simulink model "Model_GBXCluctchOpt_V5"  (R2024b)
settings: Solver=VariableStepAuto  StartTime=0.0  StopTime=552  RelTol=1e-5
undefined symbols (not defined in the file): Bdy_facCoG_C, Bdy_facTireFric_C, Bdy_lenRadiusWheel_C, Bdy_lenWheelBase_C, Bdy_lenZCoG_C, Bdy_mEquivalentJ_C, Bdy_mVeh_C, Bdy_vsqr2frc_C, Drv_kmh2gradtqDriver_C, Drv_kmh2tqDriver_C, Edr_pwr_LossMap_AXIS, Edr_pwrInverterLosses_MAP, Edr_pwrMachineLosses_MAP, Edr_rpm_InvLossMap_AXIS, Edr_rpm_MachLossMap_AXIS, Edr_rpm_MaxMinTq_AXIS, Edr_rpmMax_C, Edr_tq_MachLossMap_AXIS, Edr_tqEffMax_CUR, Env_facSlope_WLTC_CUR, Env_facSlopeBAB185_CUR, Env_facSlopeCrossCountry_CUR, Env_kmhDesBAB185_CUR, Env_kmhDesCrossCountry_CUR, Env_vVehDes_NEDC_kmh, Env_vVehDes_WLTC_kmh, Env_vVehTime_NEDC_s, Env_vVehTime_WLTC_s, Gbx_facGbxRatioRe_C, Ice_derfacLoadDecrease_MAP, Ice_derfacLoadIncrease_MAP, Ice_etaLam_CUR, Ice_facEtaCocMax_MAP, Ice_facFuelEnRich_MAP, Ice_KUMSRL_C, Ice_Lambda_AXIS, Ice_relLoad2relTqOptIgnLamOne_MAP, Ice_relLoad_AXIS, Ice_relLoad_LoadDyn_AXIS, Ice_relLoad_Max_CUR, Ice_relTq_AXIS, Ice_relTqInr2TqInr_C, Ice_relTqOptIgnLamOne2relLoad_MAP, Ice_rpm_AXIS, Ice_rpm_LoadDyn_AXIS, Ice_rpm_relLoadMax_AXIS, Ice_tqLossesIce_MAP, Pnt_capBat_C, Pnt_facSocBatOcv_AXIS, Pnt_facSocInit_C, Pnt_iBatChrgMax_C, Pnt_iBatDisChrgMax_C, Pnt_resBatInner_C, Pnt_uBatMax_C, Pnt_uBatMin_C, Pnt_uBatOcv_CUR, Vco_flgEdrExists_CFG, Vco_flgIceCluAlwClosed_CFG, Vco_flgIceExists_CFG
libraries: simulink x7, simulink_extras x6
(part 1 of 3)
settings Model: Creator=Georg  LastModifiedBy=Raj Srivastava
settings SolverCC: AlgebraicLoopSolver=TrustRegion
settings DebuggingCC: IgnoredZcDiagnostic=none  UnconnectedInputMsg=warning  UnconnectedOutputMsg=warning  UnconnectedLineMsg=warning
settings HardwareCC: ProdHWDeviceType=AMD->x86-64 (Windows64)
settings ModelReferenceCC: EnableRefExpFcnMdlSchedulingChecks=on
settings RTWCC: GPUComputeCapability=3.5  DLArmComputeVersion=19.05

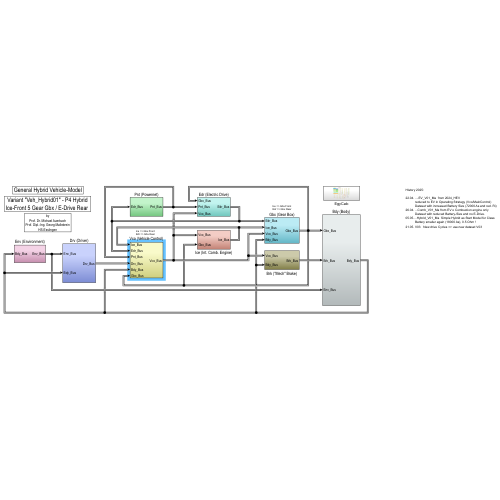
[thumbnail: Simulink's stored preview of the top-level diagram]
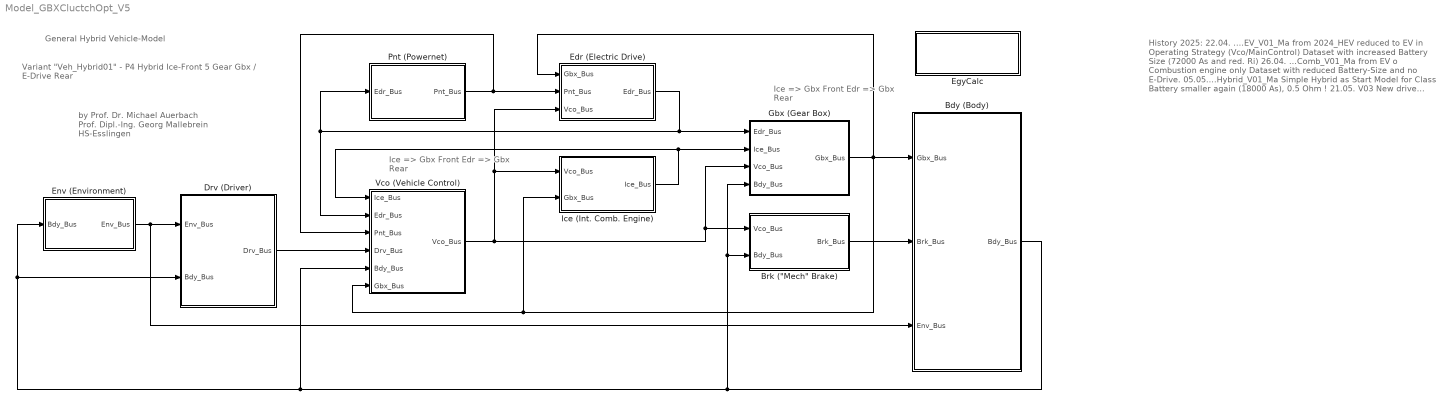
== system Model_GBXCluctchOpt_V5 ==
  note: History 2025:
      |
      | 22.04. ....EV_V01_Ma  from 2024_HEV
      |            reduced to EV in Operating Strategy (Vco/MainControl)
      |            Dataset with increased Battery Size (72000 As and red. Ri)
      | 26.04. ...Comb_V01_Ma from EV o Combustion engine only
      |            Dataset with reduced Battery-Size and no E-Drive.
      | 05.05....Hybrid_V01_Ma  Simple Hybrid as Start Model for Class
      |            Battery smaller again (18000 As), 0.5 Ohm !
      | 21.05. V03   New drive Cycles => use new dataset V03
  note: General Hybrid Vehicle-Model
  note: Ice => Gbx Front
      | Edr => Gbx Rear
  note: Ice => Gbx Front
      | Edr => Gbx Rear
  note: by
      | Prof. Dr. Michael Auerbach
      | Prof. Dipl.-Ing. Georg Mallebrein
      | HS-Esslingen
  note: Variant "Veh_Hybrid01" - P4 Hybrid
      | Ice-Front 5 Gear Gbx / E-Drive Rear
  Bdy (Body) : Subsystem
  "Brk (\"Mech\" Brake)" : Subsystem
  Drv (Driver) : Subsystem
  Edr (Electric Drive) : Subsystem
  EgyCalc : Subsystem
  Env (Environment) : Subsystem
  Gbx (Gear Box) : Subsystem
  Ice (Int. Comb. Engine) : Subsystem
  Pnt (Powernet) : Subsystem
  Vco (Vehicle Control) : Subsystem
  wires:
  Gbx (Gear Box)/1(Gbx_Bus) -> Edr (Electric Drive)/1(Gbx_Bus), Bdy (Body)/1(Gbx_Bus), Ice (Int. Comb. Engine)/2(Gbx_Bus), Vco (Vehicle Control)/6(Gbx_Bus)
  "Brk (\"Mech\" Brake)"/1(Brk_Bus) -> Bdy (Body)/2(Brk_Bus)
  Pnt (Powernet)/1(Pnt_Bus) -> Edr (Electric Drive)/2(Pnt_Bus), Vco (Vehicle Control)/3(Pnt_Bus)
  Edr (Electric Drive)/1(Edr_Bus) -> Vco (Vehicle Control)/2(Edr_Bus), Pnt (Powernet)/1(Edr_Bus), Gbx (Gear Box)/1(Edr_Bus)
  Ice (Int. Comb. Engine)/1(Ice_Bus) -> Vco (Vehicle Control)/1(Ice_Bus), Gbx (Gear Box)/2(Ice_Bus)
  Vco (Vehicle Control)/1(Vco_Bus) -> Edr (Electric Drive)/3(Vco_Bus), Ice (Int. Comb. Engine)/1(Vco_Bus), Gbx (Gear Box)/3(Vco_Bus), "Brk (\"Mech\" Brake)"/1(Vco_Bus)
  Drv (Driver)/1(Drv_Bus) -> Vco (Vehicle Control)/4(Drv_Bus)
  Env (Environment)/1(Env_Bus) -> Bdy (Body)/3(Env_Bus), Drv (Driver)/1(Env_Bus)
  Bdy (Body)/1(Bdy_Bus) -> Env (Environment)/1(Bdy_Bus), Drv (Driver)/2(Bdy_Bus), Vco (Vehicle Control)/5(Bdy_Bus), "Brk (\"Mech\" Brake)"/2(Bdy_Bus), Gbx (Gear Box)/4(Bdy_Bus)

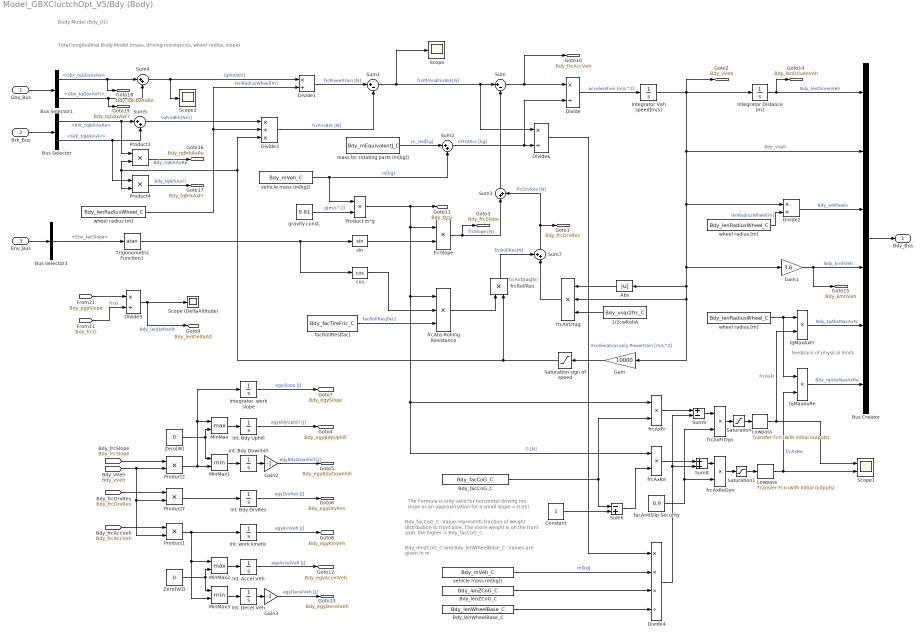
== system Model_GBXCluctchOpt_V5/Bdy (Body) ==
  note: feedback of physical limits
  note: Bdy_facCoG_C: Value represents fraction of weight distribution to front axle. The more weight is on the front axle, the higher is Bdy_facCoG_C.
  note: Total longitudinal Body Model (mass, driving resistances, wheel radius, slope)
  note: Bdy_lenZCoG_C and Bdy_lenWheelBase_C: Values are given in m
  note: The Formula is only valid for horizontal driving (no slope or an approximation for a small slope < 0.05)
  note: Body Model (Bdy_01)
  Gbx_Bus : Inport
  Brk_Bus : Inport  Port=2
  Env_Bus : Inport  Port=3
  " wheel radius [m]  " : Constant  Value=Bdy_lenRadiusWheel_C
  1/2cwRohA : Constant  Value=Bdy_vsqr2frc_C
  Abs : Abs  SaturateOnIntegerOverflow=off
  Bdy_facCoG_C : Constant  Value=Bdy_facCoG_C
  Bdy_lenWheelBase_C : Constant  Value=Bdy_lenWheelBase_C
  Bdy_lenZCoG_C : Constant  Value=Bdy_lenZCoG_C
  Bus Creator : BusCreator  Inputs=6
  Bus Selector : BusSelector  OutputSignals=Brk_tqBrkAxRe,Brk_tqBrkAxFr
  Bus Selector1 : BusSelector  OutputSignals=Gbx_tqGbxAxRe,Gbx_tqGbxAxFr
  Bus Selector3 : BusSelector  OutputSignals=Env_facSlope
  Constant : Constant
  Divide{,1..2,5..6} (5 alike) : Product  Inputs=*/
  Divide3 : Product  Inputs=*/*
  Divide4 : Product  Inputs=***/
  Gain : Gain  Gain=10000
  Gain1 : Gain  Gain=3.6
  Gain2 : Gain  Gain=-1
  Gain3 : Gain  Gain=-1
  Int. Accel Veh : Integrator
  Int. Bdy Downhill : Integrator
  Int. Bdy DrvRes : Integrator
  Int. Bdy Uphill : Integrator
  Int. Decel Veh : Integrator
  Int. work kinetic : Integrator
  Integrator Distance [m] : Integrator  InitialCondition=1E-10
  Integrator Veh speed[m/s] : Integrator
  Integrator  work slope : Integrator
  Lowpass : simulink_extras/Additional Linear/Transfer Fcn (with initial outputs)  N=[1]  D=[0.000001 1]  Y0=1  U0=0
  "Lowpass " : simulink_extras/Additional Linear/Transfer Fcn (with initial outputs)  N=[1]  D=[0.000001 1]  Y0=1  U0=0
  MinMax : MinMax  Function=max  Inputs=2  ZeroCross=off
  MinMax1 : MinMax  Inputs=2  ZeroCross=off
  MinMax2 : MinMax  Function=max  Inputs=2  ZeroCross=off
  MinMax3 : MinMax  Inputs=2  ZeroCross=off
  Product m*g : Product
  Product{1..4,7} (5 alike) : Product
  Saturation : Saturate  UpperLimit=inf  LowerLimit=0
  Saturation sign of speed : Saturate  UpperLimit=1  LowerLimit=-1
  Saturation1 : Saturate  UpperLimit=inf  LowerLimit=0
  Scope : Scope
  "Scope (DeltaAltitude) " : Scope
  Scope1 : Scope  NumInputPorts=2
  Scope2 : Scope
  Sum : Sum  Inputs=|+-
  Sum1 : Sum  Inputs=|+-
  Sum{2..5} (4 alike) : Sum  Inputs=|++
  Sum6 : Sum  Inputs=-+
  Sum7 : Sum  Inputs=++|
  Sum8 : Sum
  Sum9 : Sum  Inputs=+-
  Trigonometric Function1 : Trigonometry  Operator=atan
  Zero[W] : Constant  Value=0
  Zero[W]1 : Constant  Value=0
  cos : Trigonometry  Operator=cos
  facAntiSlip Security : Constant  Value=0.9
  facRollRes[fac] : Constant  Value=Bdy_facTireFric_C
  frcAbs Rolling Resistance : Product  Inputs=3
  frcAirDrag : Product  Inputs=3
  frcAxFr : Product
  frcAxFrDyn : Product
  frcAxRe : Product
  frcAxReDyn : Product
  frcRollRes : Product
  frcSlope : Product
  gravity const. : Constant  Value=9.81
  mass for rotating parts (m[kg]) : Constant  Value=Bdy_mEquivalentJ_C
  sin : Trigonometry
  tqMaxAxFr : Product
  tqMaxAxRe : Product
  vehicle mass (m[kg]) : Constant  Value=Bdy_mVeh_C
  "vehicle mass (m[kg]) " : Constant  Value=Bdy_mVeh_C
  wheel radius [m] : Constant  Value=Bdy_lenRadiusWheel_C
  "wheel radius [m] " : Constant  Value=Bdy_lenRadiusWheel_C
  Bdy_Bus : Outport  VectorParamsAs1DForOutWhenUnconnected=off
  tag scope: Bdy_egyAccelVeh=global, Bdy_egyBdyDownhill=global, Bdy_egyBdyUphill=global, Bdy_egyDecelVeh=global, Bdy_egyDrvRes=global, Bdy_egyKinVeh=global, Bdy_egySlope=global, Bdy_frcAccVeh=global, Bdy_frcDrvRes=global, Bdy_frcG=global, Bdy_frcSlope=global, Bdy_kmhVeh=global, Bdy_lenDeltaAlt=global, Bdy_lenDrivenVeh=global, Bdy_tqBrkAxFr=global, Bdy_tqBrkAxRe=global, Bdy_tqGbxAxFr=global, Bdy_tqGbxAxRe=global, Bdy_vVeh=global
  wires:
  Bus Creator/1 -> Bdy_Bus/1
  Gbx_Bus/1 -> Bus Selector1/1
  Brk_Bus/1 -> Bus Selector/1
  Bus Selector/1 -> Sum5/1, Product3/1  "<Brk_tqBrkAxRe>"
  Bus Selector/2 -> Product4/1, Sum5/2  "<Brk_tqBrkAxFr>"
  Divide2/1 -> Bus Creator/3  "Bdy_wWheels"
  Bus Selector1/1 -> [Bdy_tqGbxAxRe], Sum4/1  "<Gbx_tqGbxAxRe>"
  Bus Selector1/2 -> [Bdy_tqGbxAxFr], Sum4/2  "<Gbx_tqGbxAxFr>"
  Env_Bus/1 -> Bus Selector3/1
  Bus Selector3/1 -> Trigonometric Function1/1  "<Env_facSlope>"
  Integrator Distance [m]/1 -> [Bdy_lenDrivenVeh], Bus Creator/1  "Bdy_lenDrivenVeh"
  Integrator Veh speed[m/s]/1 -> [Bdy_vVeh], Integrator Distance [m]/1, Gain1/1, Abs/1, frcAirDrag/2, Gain/1, Divide2/1, Bus Creator/2  "Bdy_vVeh"
  frcAirDrag/1 -> Sum7/2  "frcAirDrag[N]"
  1/2cwRohA/1 -> frcAirDrag/3
  frcRollRes/1 -> Sum7/1  "frcRollRes[N]"
  Divide/1 -> Integrator Veh speed[m/s]/1  "acceleration [m/s^2]"
  sin/1 -> frcSlope/2
  cos/1 -> frcAbs Rolling Resistance/2
  Gain/1 -> Saturation sign of speed/1
  Divide1/1 -> Sum1/1  "frcPowertrain [N]"
  Saturation sign of speed/1 -> Product3/2, Product4/2, Divide3/3, frcRollRes/2
  Sum1/1 -> Scope/1, Divide6/1, Sum/1  "frcPtrAndFricBrk[N]"
  Sum5/1 -> Divide3/1  "tqFricBrk[Nm]"
  Sum2/1 -> Divide6/2, Divide/2  "mTotAcc [kg]"
  Sum7/1 -> [Bdy_frcDrvRes], Sum3/2  "frcDrvRes [N]"
  Product m*g/1 -> [Bdy_frcG], frcSlope/1, frcAxRe/1, frcAxFr/1, frcAbs Rolling Resistance/1  "G [N]"
  frcAbs Rolling Resistance/1 -> frcRollRes/1
  Divide3/1 -> Sum1/2  "frcFricBrk [N]"
  Abs/1 -> frcAirDrag/1
  mass for rotating parts (m[kg])/1 -> Sum2/1  "m_red[kg]"
  frcSlope/1 -> [Bdy_frcSlope], Sum3/1  "frcSlope [N]"
  Sum3/1 -> Sum/2
  facRollRes[fac]/1 -> frcAbs Rolling Resistance/3  "facRollRes[fac]"
  Trigonometric Function1/1 -> cos/1, sin/1
  wheel radius [m]/1 -> Divide1/2, Divide3/2  "lenRadiusWheel[m]"
  Sum4/1 -> Scope2/1, Divide1/1  "tqPtr[Nm]"
  vehicle mass (m[kg])/1 -> Sum2/2, Product m*g/1  "m[kg]"
  gravity const./1 -> Product m*g/2  "g[m/s^2]"
  Sum/1 -> [Bdy_frcAccVeh], Divide/1
  "wheel radius [m] "/1 -> Divide2/2  "lenRadiusWheel[m]"
  Gain1/1 -> [Bdy_kmhVeh], Bus Creator/4  "Bdy_kmhVeh"
  tqMaxAxFr/1 -> Bus Creator/5  "Bdy_tqAbsMaxAxFr"
  tqMaxAxRe/1 -> Bus Creator/6  "Bdy_tqAbsMaxAxRe"
  " wheel radius [m]  "/1 -> tqMaxAxFr/1, tqMaxAxRe/1
  frcAxFr/1 -> Sum9/1
  frcAxRe/1 -> Sum8/1
  "Lowpass "/1 -> tqMaxAxRe/2, Scope1/2  "frcAxRe"
  Lowpass/1 -> tqMaxAxFr/2, Scope1/1  "frcAxFr"
  Sum6/1 -> frcAxRe/2
  Bdy_facCoG_C/1 -> frcAxFr/2, Sum6/1
  Constant/1 -> Sum6/2
  Bdy_lenZCoG_C/1 -> Divide4/3
  Bdy_lenWheelBase_C/1 -> Divide4/4
  Sum8/1 -> frcAxReDyn/1
  Sum9/1 -> frcAxFrDyn/1
  "vehicle mass (m[kg]) "/1 -> Divide4/2  "m[kg]"
  facAntiSlip Security/1 -> frcAxReDyn/2, frcAxFrDyn/2
  frcAxFrDyn/1 -> Saturation/1
  Saturation/1 -> Lowpass/1
  frcAxReDyn/1 -> Saturation1/1
  Saturation1/1 -> "Lowpass "/1
  Zero[W]/1 -> MinMax1/1, MinMax/2
  Int. Bdy Downhill/1 -> Gain2/1
  Int. Bdy DrvRes/1 -> [Bdy_egyDrvRes]  "egyDrvRes [J]"
  Int. Bdy Uphill/1 -> [Bdy_egyBdyUphill]  "egyBdyUphill [J]"
  MinMax1/1 -> Int. Bdy Downhill/1
  Product2/1 -> Integrator  work slope/1, MinMax/1, MinMax1/2
  MinMax/1 -> Int. Bdy Uphill/1
  Product7/1 -> Int. Bdy DrvRes/1
  Gain2/1 -> [Bdy_egyBdyDownhill]  "egyBdyDownhill [J]"
  [Bdy_vVeh] -> Product1/2, Product7/2, Product2/2
  [Bdy_frcDrvRes] -> Product7/1
  [Bdy_frcSlope] -> Product2/1
  Integrator  work slope/1 -> [Bdy_egySlope]  "egySlope [J]"
  [Bdy_frcG] -> Divide5/2  "frcG"
  Divide5/1 -> [Bdy_lenDeltaAlt], "Scope (DeltaAltitude) "/1  "Bdy_lenDeltaAlt"
  [Bdy_egySlope] -> Divide5/1
  Int. work kinetic/1 -> [Bdy_egyKinVeh]  "egyKinVeh [J]"
  Product1/1 -> MinMax3/2, MinMax2/1, Int. work kinetic/1
  [Bdy_frcAccVeh] -> Product1/1
  Int. Accel Veh/1 -> [Bdy_egyAccelVeh]  "egyAccelVeh [J]"
  MinMax3/1 -> Int. Decel Veh/1
  Zero[W]1/1 -> MinMax3/1, MinMax2/2
  Gain3/1 -> [Bdy_egyDecelVeh]  "egyDecelVeh [J]"
  MinMax2/1 -> Int. Accel Veh/1
  Int. Decel Veh/1 -> Gain3/1
  Product3/1 -> [Bdy_tqBrkAxRe]  "Bdy_tqBrkAxRe"
  Product4/1 -> [Bdy_tqBrkAxFr]  "Bdy_tqBrkAxFr"
  Divide6/1 -> Divide4/1  "Acceleration only Powertrain [m/s^2]"
  Divide4/1 -> Sum8/2, Sum9/2

== system Model_GBXCluctchOpt_V5/Brk ("Mech" Brake) ==
  note: Mechanical Brake Model (Brk_01)
      | (both Axles)
  note: Info:
      | tq here is wheel axle based
  note: - very simple here, but a dynamik brake is not needed here
  Vco_Bus : Inport
  Bdy_Bus : Inport  Port=2
  Bus Creator : BusCreator  Inputs=2
  Bus Selector1 : BusSelector  OutputSignals=BrkCtrl_tqBrkAxReDes,BrkCtrl_tqBrkAxFrDes
  Bus Selector2 : BusSelector  OutputSignals=Bdy_wWheels
  Gain : Gain
  Gain1 : Gain
  Int. Brk LossesFr : Integrator
  Int. Brk LossesRe : Integrator
  Product1 : Product
  Product7 : Product
  Scope2 : Scope
  Brk_Bus : Outport  VectorParamsAs1DForOutWhenUnconnected=off
  tag scope: Brk_egyBrkLossesFr=global, Brk_egyBrkLossesRe=global
  wires:
  Vco_Bus/1 -> Bus Selector1/1
  Bus Selector1/1 -> Gain/1  "<BrkCtrl_tqBrkAxReDes>"
  Bus Selector1/2 -> Gain1/1  "<BrkCtrl_tqBrkAxFrDes>"
  Bus Creator/1 -> Brk_Bus/1
  Gain/1 -> Product7/1, Bus Creator/1  "Brk_tqBrkAxRe"
  Gain1/1 -> Scope2/1, Bus Creator/2, Product1/1  "Brk_tqBrkAxFr"
  Bdy_Bus/1 -> Bus Selector2/1
  Bus Selector2/1 -> Product1/2, Product7/2  "<Bdy_wWheels>"
  Int. Brk LossesRe/1 -> [Brk_egyBrkLossesRe]  "egyBrkLossesRe [J]"
  Product7/1 -> Int. Brk LossesRe/1
  Int. Brk LossesFr/1 -> [Brk_egyBrkLossesFr]  "egyBrkLossesFr [J]"
  Product1/1 -> Int. Brk LossesFr/1

== system Model_GBXCluctchOpt_V5/Drv (Driver) ==
  note: Desired speed limited with max. speed of E-Drive
  note: Driver Model for total EV-Model (Drv_01)
  note: Info:
      | tq here is wheel axle based
  Env_Bus : Inport
  Bdy_Bus : Inport  Port=2
  Bus Creator : BusCreator  Inputs=2
  Bus Selector : BusSelector  OutputSignals=Env_kmhVehDes
  Bus Selector1 : BusSelector  OutputSignals=Bdy_kmhVeh
  Drv_kmh2gradtqDriver_C : Gain  Gain=Drv_kmh2gradtqDriver_C
  Drv_kmh2tqDriver_C : Gain  Gain=Drv_kmh2tqDriver_C
  Feedback I-Part at v=0 : Lookup_n-D  NumberOfTableDimensions=1  BreakpointsForDimension1="[-1 -0.0001  0  0.0001  1]"  Table="[0 0  1  0  0]"  InternalRulePriority=Speed  RndMeth=Simplest
  Gain : Gain
  Gain1 : Gain  Gain=0.005
  Integrator : Integrator  LimitOutput=on  UpperSaturationLimit=1200  LowerSaturationLimit=-1200
  LowPass4Solver : TransferFcn  Denominator=[0.0001 1]
  MinMax : MinMax  Inputs=2
  Mux : Mux  Inputs=2
  Product : Product
  Saturation : Saturate  UpperLimit=3000  LowerLimit=-5000
  Saturation1 : Saturate  UpperLimit=3000  LowerLimit=-5000
  Scope Ctrl. : Scope  NumInputPorts=2
  Scope Ctrl.1 : Scope  NumInputPorts=2
  Scope kmh : Scope
  Sum : Sum  Inputs=|+-
  Sum1 : Sum  Inputs=|++
  Sum2 : Sum  Inputs=|+-
  v_maxKmhEdr : Constant  Value=Edr_rpmMax_C*pi()/30/Gbx_facGbxRatioRe_C*Bdy_lenRadiusWheel_C*3.6
  Drv_Bus : Outport  VectorParamsAs1DForOutWhenUnconnected=off
  wires:
  Mux/1 -> Scope kmh/1
  Bus Selector1/1 -> Feedback I-Part at v=0/1, Sum/2, Mux/2  "<Bdy_kmhVeh>"
  Integrator/1 -> Gain1/1, Sum1/2, Scope Ctrl./2  "Drv_tqICtrlDrv[Nm]"
  Drv_kmh2gradtqDriver_C/1 -> Integrator/1
  Saturation/1 -> Sum1/1, Scope Ctrl./1  "Drv_tqPCtrlDrv[Nm]"
  Bus Selector/1 -> MinMax/2  "<Env_kmhVehDes>"
  Bus Creator/1 -> Drv_Bus/1
  Bdy_Bus/1 -> Bus Selector1/1
  Env_Bus/1 -> Bus Selector/1
  Drv_kmh2tqDriver_C/1 -> LowPass4Solver/1
  MinMax/1 -> Gain/1, Sum/1, Mux/1  "Env_kmhVehDesLim"
  Gain/1 -> Bus Creator/2  "Drv_kmhVehDesLim"
  Saturation1/1 -> Scope Ctrl.1/2, Bus Creator/1  "Drv_tqDrvWheelAxDes"
  Sum/1 -> Sum2/1, Drv_kmh2tqDriver_C/1
  Sum2/1 -> Drv_kmh2gradtqDriver_C/1
  Product/1 -> Sum2/2
  Gain1/1 -> Product/2  "Drv_kmhVehDesLim"
  Feedback I-Part at v=0/1 -> Product/1
  v_maxKmhEdr/1 -> MinMax/1
  LowPass4Solver/1 -> Saturation/1
  Sum1/1 -> Scope Ctrl.1/1, Saturation1/1  "tqDrvWheelAxDesUnlim"

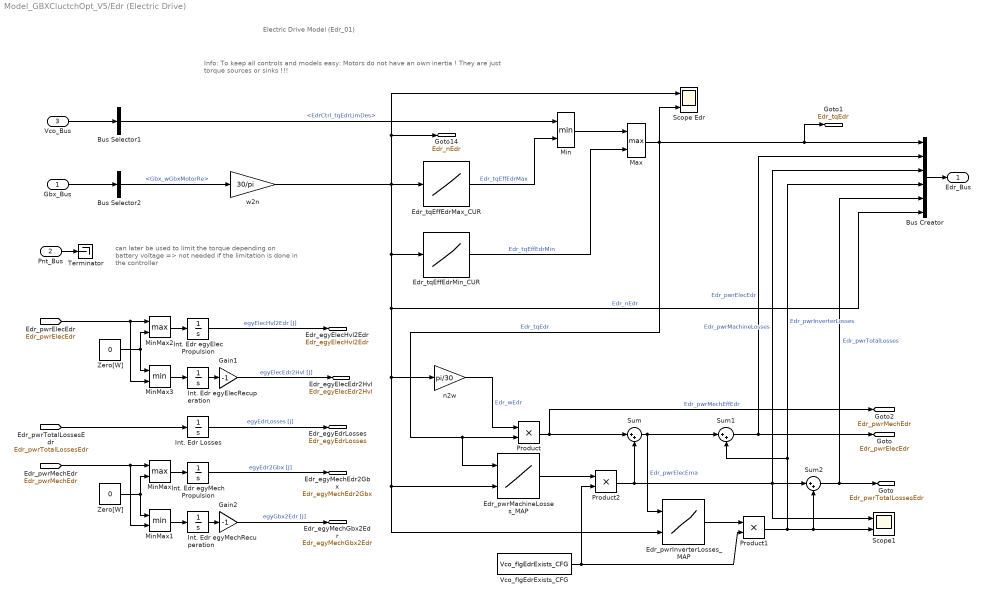
== system Model_GBXCluctchOpt_V5/Edr (Electric Drive) ==
  note: Info: To keep all controls and models easy: Motors do not have an own inertia !
      | They are just torque sources or sinks !!!
  note: can later be used to limit the torque
      | depending on battery voltage
      | => not needed if the limitation is done in the controller
  note: Electric Drive Model (Edr_01)
  Gbx_Bus : Inport
  Pnt_Bus : Inport  Port=2
  Vco_Bus : Inport  Port=3
  Bus Creator : BusCreator  Inputs=6
  Bus Selector1 : BusSelector  OutputSignals=EdrCtrl_tqEdrLimDes
  Bus Selector2 : BusSelector  OutputSignals=Gbx_wGbxMotorRe
  Edr_pwrInverterLosses_MAP : Lookup_n-D  BreakpointsForDimension1=Edr_pwr_LossMap_AXIS  BreakpointsForDimension2=Edr_rpm_InvLossMap_AXIS  Table=Edr_pwrInverterLosses_MAP  ExtrapMethod=Clip  UseLastTableValue=on  InternalRulePriority=Speed  RndMeth=Simplest
      settings: InputPortMap=u0,u1
  Edr_pwrMachineLosses_MAP : Lookup_n-D  BreakpointsForDimension1=Edr_tq_MachLossMap_AXIS  BreakpointsForDimension2=Edr_rpm_MachLossMap_AXIS  Table=Edr_pwrMachineLosses_MAP  ExtrapMethod=Clip  UseLastTableValue=on  InternalRulePriority=Speed  RndMeth=Simplest
      settings: InputPortMap=u0,u1
  Edr_tqEffEdrMax_CUR : Lookup_n-D  NumberOfTableDimensions=1  BreakpointsForDimension1=Edr_rpm_MaxMinTq_AXIS  Table=Edr_tqEffMax_CUR  ExtrapMethod=Clip  InternalRulePriority=Speed  RndMeth=Simplest
  Edr_tqEffEdrMin_CUR : Lookup_n-D  NumberOfTableDimensions=1  BreakpointsForDimension1=Edr_rpm_MaxMinTq_AXIS  Table=-Edr_tqEffMax_CUR  ExtrapMethod=Clip  InternalRulePriority=Speed  RndMeth=Simplest
  Gain1 : Gain  Gain=-1
  Gain2 : Gain  Gain=-1
  Int. Edr Losses : Integrator
  Int. Edr egyElec Propulsion : Integrator
  Int. Edr egyElecRecuperation : Integrator
  Int. Edr egyMech Propulsion : Integrator
  Int. Edr egyMechRecuperation : Integrator
  Max : MinMax  Function=max  Inputs=2
  Min : MinMax  Inputs=2
  MinMax : MinMax  Function=max  Inputs=2  ZeroCross=off
  MinMax1 : MinMax  Inputs=2  ZeroCross=off
  MinMax2 : MinMax  Function=max  Inputs=2  ZeroCross=off
  MinMax3 : MinMax  Inputs=2  ZeroCross=off
  Product : Product
  Product1 : Product
  Product2 : Product
  Scope Edr : Scope  NumInputPorts=2
  Scope1 : Scope  NumInputPorts=2
  Sum : Sum  Inputs=|++
  Sum1 : Sum  Inputs=|++
  Sum2 : Sum  Inputs=|++
  Terminator : Terminator
  Vco_flgEdrExists_CFG : Constant  Value=Vco_flgEdrExists_CFG
  Zero[W] : Constant  Value=0
  "Zero[W] " : Constant  Value=0
  n2w : Gain  Gain=pi/30
  w2n : Gain  Gain=30/pi
  Edr_Bus : Outport  VectorParamsAs1DForOutWhenUnconnected=off
  tag scope: Edr_egyEdrLosses=global, Edr_egyElecEdr2Hvl=global, Edr_egyElecHvl2Edr=global, Edr_egyMechEdr2Gbx=global, Edr_egyMechGbx2Edr=global, Edr_nEdr=global, Edr_pwrElecEdr=global, Edr_pwrMechEdr=global, Edr_pwrTotalLossesEdr=global, Edr_tqEdr=global
  wires:
  Vco_Bus/1 -> Bus Selector1/1
  Bus Creator/1 -> Edr_Bus/1
  Bus Selector1/1 -> Min/1  "<EdrCtrl_tqEdrLimDes>"
  Max/1 -> [Edr_tqEdr], Bus Creator/1, Product/2, Edr_pwrMachineLosses_MAP/1, Scope Edr/2  "Edr_tqEdr"
  Min/1 -> Max/1
  Edr_tqEffEdrMin_CUR/1 -> Max/2  "Edr_tqEffEdrMin"
  Product1/1 -> Sum1/2, Bus Creator/4, Scope1/2, Sum2/2  "Edr_pwrInverterLosses"
  Sum/1 -> Sum1/1, Edr_pwrInverterLosses_MAP/1  "Edr_pwrElecEma"
  n2w/1 -> Product/1  "Edr_wEdr"
  Edr_tqEffEdrMax_CUR/1 -> Min/2  "Edr_tqEffEdrMax"
  Product/1 -> Sum/1, [Edr_pwrMechEdr]  "Edr_pwrMechEffEdr"
  Product2/1 -> Bus Creator/3, Sum2/1, Scope1/1, Sum/2  "Edr_pwrMachineLosses"
  Sum2/1 -> [Edr_pwrTotalLossesEdr], Bus Creator/5  "Edr_pwrTotalLosses"
  w2n/1 -> Edr_pwrInverterLosses_MAP/2, Edr_pwrMachineLosses_MAP/2, n2w/1, Bus Creator/6, Edr_tqEffEdrMin_CUR/1, Edr_tqEffEdrMax_CUR/1, [Edr_nEdr], Scope Edr/1  "Edr_nEdr"
  Gbx_Bus/1 -> Bus Selector2/1
  Bus Selector2/1 -> w2n/1  "<Gbx_wGbxMotorRe>"
  Sum1/1 -> [Edr_pwrElecEdr], Bus Creator/2  "Edr_pwrElecEdr"
  [Edr_pwrElecEdr] -> MinMax2/1, MinMax3/2
  Int. Edr egyElecRecuperation/1 -> Gain1/1
  MinMax3/1 -> Int. Edr egyElecRecuperation/1
  "Zero[W] "/1 -> MinMax3/1, MinMax2/2
  Int. Edr egyElec Propulsion/1 -> [Edr_egyElecHvl2Edr]  "egyElecHvl2Edr [J]"
  MinMax2/1 -> Int. Edr egyElec Propulsion/1
  Gain1/1 -> [Edr_egyElecEdr2Hvl]  "egyElecEdr2Hvl [J]"
  [Edr_pwrTotalLossesEdr] -> Int. Edr Losses/1
  Zero[W]/1 -> MinMax1/1, MinMax/2
  Int. Edr egyMech Propulsion/1 -> [Edr_egyMechEdr2Gbx]  "egyEdr2Gbx [J]"
  MinMax/1 -> Int. Edr egyMech Propulsion/1
  [Edr_pwrMechEdr] -> MinMax/1, MinMax1/2
  MinMax1/1 -> Int. Edr egyMechRecuperation/1
  Gain2/1 -> [Edr_egyMechGbx2Edr]  "egyGbx2Edr [J]"
  Int. Edr egyMechRecuperation/1 -> Gain2/1
  Int. Edr Losses/1 -> [Edr_egyEdrLosses]  "egyEdrLosses [J]"
  Pnt_Bus/1 -> Terminator/1
  Edr_pwrInverterLosses_MAP/1 -> Product1/1
  Vco_flgEdrExists_CFG/1 -> Product1/2, Product2/2
  Edr_pwrMachineLosses_MAP/1 -> Product2/1

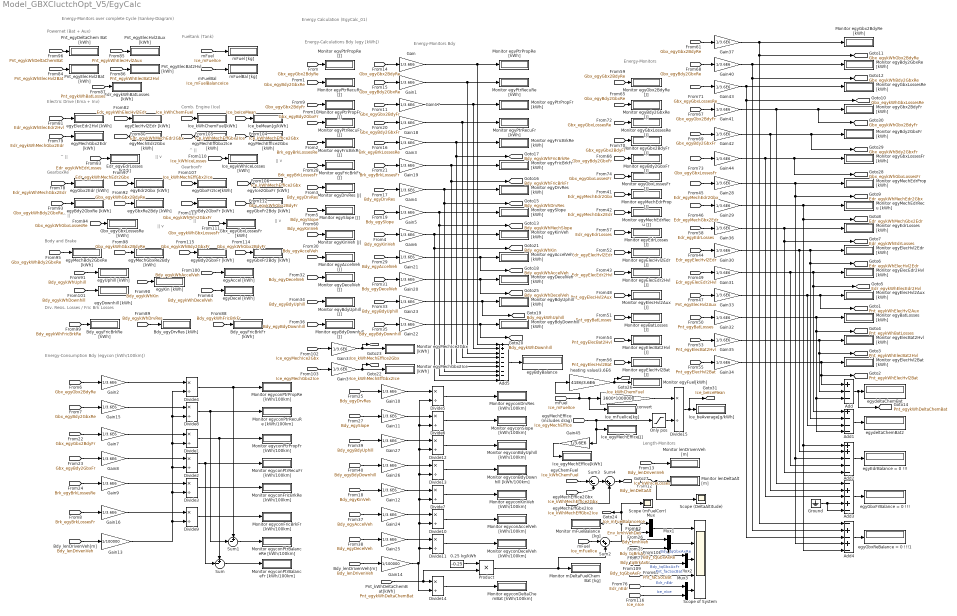
== system Model_GBXCluctchOpt_V5/EgyCalc ==
  note: Energy-Consumption Bdy (egycon [kWh/100km])
  note: Energy-Monitors Bdy
  note: Length-Monitors
  note: Energy-Calculations Bdy (egy [kWh])
  note: Energy-Monitors
  note: Energy Calculation (EgyCalc_01)
  note: ||
      | v
  note: Powernet (Bat + Aux)
  note: GearboxRe
  note: ^
      | ||
  note: ||
      | v
  note: ^
      | ||
  note: Energy-Monitors over complete Cycle
      | (Sankey-Diagram)
  note: Electric Drive (Ema + Inv)
  note: Drv. Resis. Losses / Fric Brk Losses
  note: Body and Brake
  note: Comb. Engine (Ice)
  note: Fueltank (Tank)
  note: ^
      | ||
  note: ||
      | v
  note: GearboxFr
  note: ^
      | ||
  note: ||
      | v
  0.25 kg/kWh : Constant  Value=-0.25
  Add : Sum  Inputs=+--
  Add1 : Sum  Inputs=+---
  Add2 : Sum  Inputs=++---
  Add3 : Sum  Inputs=-+-+-
  Add4 : Sum  Inputs=-+-+-
  Add5 : Sum  Inputs=++-------
  Bdy_egyDrvRes [kWh] : Display
      settings: Format=bank
  Bdy_egyFricBrkFr [kWh] : Display
      settings: Format=bank
  Bdy_egyFricBrkRe [kWh] : Display
      settings: Format=bank
  Divide{1..15} (15 alike) : Product  Inputs=*/
  Edr_egyEdrLosses [kWh] : Display
      settings: Format=bank
  Edr_egykWhBatLosses [kWh] : Display
      settings: Format=bank
  Gain{,1..12,15..45} (44 alike) : Gain  Gain=1/3.6E6
  Gain13 : Gain  Gain=1/100000
  Gain14 : Gain  Gain=1/100000
  Gbx_egyGbxLossesFr [kWh] : Display
      settings: Format=bank
  Gbx_egyGbxLossesRe [kWh] : Display
      settings: Format=bank
  Ground : Ground
  Ice_beAverage[g/kWh] : Display
  Ice_beMean[g/kWh] : Display
      settings: Format=bank
  Ice_egyMechEffIce[J] : Display
  Ice_egyMechEffIce[kWh] : Display
  Ice_egykWhIceLosses [kWh] : Display
      settings: Format=bank
  Ice_kWhChemFuel[kWh] : Display
      settings: Format=bank
  Ice_mFuelIce[kg] : Display
  Monitor egyAccelVeh [J] : Display
      settings: Format=short_e
  Monitor egyAccelVeh [kWh] : Display
  Monitor egyBatLosses [J] : Display
      settings: Format=short_e
  Monitor egyBatLosses [kWh] : Display
  Monitor egyBdy2GbxFr [J] : Display
      settings: Format=short_e
  Monitor egyBdy2GbxFr [kWh] : Display
  Monitor egyBdy2GbxRe [J] : Display
      settings: Format=short_e
  Monitor egyBdy2GbxRe [kWh] : Display
  Monitor egyBdyDownhill [J] : Display
      settings: Format=short_e
  Monitor egyBdyDownhill [kWh] : Display
  Monitor egyBdyUphill [J] : Display
      settings: Format=short_e
  Monitor egyBdyUphill [kWh] : Display
  Monitor egyDecelVeh [J] : Display
      settings: Format=short_e
  Monitor egyDecelVeh [kWh] : Display
  Monitor egyDrvRes [J] : Display
      settings: Format=short_e
  Monitor egyDrvRes [kWh] : Display
  Monitor egyEdrLosses [J] : Display
      settings: Format=short_e
  Monitor egyEdrLosses [kWh] : Display
  Monitor egyElecBat2Hvl [J] : Display
      settings: Format=short_e
  Monitor egyElecBat2Hvl [kWh] : Display
  Monitor egyElecEdr2Hvl [J] : Display
      settings: Format=short_e
  Monitor egyElecEdr2Hvl [kWh] : Display
  Monitor egyElecHvl2Aux [J] : Display
      settings: Format=short_e
  Monitor egyElecHvl2Aux [kWh] : Display
  Monitor egyElecHvl2Bat [J] : Display
      settings: Format=short_e
  Monitor egyElecHvl2Bat [kWh] : Display
  Monitor egyElecHvl2Edr [J] : Display
      settings: Format=short_e
  Monitor egyElecHvl2Edr [kWh] : Display
  Monitor egyFricBrkFr [J] : Display
      settings: Format=short_e
  Monitor egyFricBrkFr [kWh] : Display
  Monitor egyFricBrkRe [J] : Display
      settings: Format=short_e
  Monitor egyFricBrkRe [kWh] : Display
  Monitor egyFuel[kWh] : Display
      settings: Format=bank
  Monitor egyGbx2BdyFr [J] : Display
      settings: Format=short_e
  Monitor egyGbx2BdyFr [kWh] : Display
  Monitor egyGbx2BdyRe [J] : Display
      settings: Format=short_e
  Monitor egyGbx2BdyRe [kWh] : Display
  Monitor egyGbxLossesFr [J] : Display
      settings: Format=short_e
  Monitor egyGbxLossesFr [kWh] : Display
  Monitor egyGbxLossesRe [J] : Display
      settings: Format=short_e
  Monitor egyGbxLossesRe [kWh] : Display
  Monitor egyKinVeh [J] : Display
      settings: Format=short_e
  Monitor egyKinVeh [kWh] : Display
      settings: Format=bank
  Monitor egyMechEdrProp [J] : Display
      settings: Format=short_e
  Monitor egyMechEdrProp [kWh] : Display
  Monitor egyMechEdrRecu [J] : Display
      settings: Format=short_e
  Monitor egyMechEdrRecu [kWh] : Display
  Monitor egyMechGbx2Ice [kWh] : Display
  Monitor egyMechIce2Gbx [kWh] : Display
  Monitor egyPtrPropFr [J] : Display
      settings: Format=short_e
  Monitor egyPtrPropFr [kWh] : Display
  Monitor egyPtrPropRe [J] : Display
      settings: Format=short_e
  Monitor egyPtrPropRe [kWh] : Display
  Monitor egyPtrRecuFr [J] : Display
      settings: Format=short_e
  Monitor egyPtrRecuFr [kWh] : Display
  Monitor egyPtrRecuRe [J] : Display
      settings: Format=short_e
  Monitor egyPtrRecuRe [kWh] : Display
  Monitor egySlope [J] : Display
      settings: Format=short_e
  Monitor egySlope [kWh] : Display
  Monitor egyconAccelVeh [kWh/100km] : Display
      settings: Format=bank
  Monitor egyconBdyDownhill [kWh/100km] : Display
      settings: Format=bank
  Monitor egyconBdyUphill [kWh/100km] : Display
      settings: Format=bank
  Monitor egyconDecelVeh [kWh/100km] : Display
      settings: Format=bank
  Monitor egyconDeltaChemBat [kWh/100km] : Display
      settings: Format=bank
  Monitor egyconDrvRes [kWh/100km] : Display
      settings: Format=bank
  Monitor egyconFricBrkFr [kWh/100km] : Display
      settings: Format=bank
  Monitor egyconFricBrkRe [kWh/100km] : Display
      settings: Format=bank
  Monitor egyconKinVeh [kWh/100km] : Display
      settings: Format=bank
  Monitor egyconPtrBalanceFr [kWh/100km] : Display
      settings: Format=bank
  Monitor egyconPtrBalanceRe [kWh/100km] : Display
      settings: Format=bank
  Monitor egyconPtrPropFr [kWh/100km] : Display
      settings: Format=bank
  Monitor egyconPtrPropRe [kWh/100km] : Display
      settings: Format=bank
  Monitor egyconPtrRecuFr [kWh/100km] : Display
      settings: Format=bank
  Monitor egyconPtrRecuRe [kWh/100km] : Display
      settings: Format=bank
  Monitor egyconSlope [kWh/100km] : Display
      settings: Format=bank
  Monitor lenDeltaAlt [m] : Display
      settings: Format=bank
  Monitor lenDrivenVeh [m] : Display
      settings: Format=bank
  Monitor mDeltaFuelChemBat [kg] : Display
      settings: Format=bank
  Monitor mFuelBalance [kg] : Display
      settings: Format=bank
  Mux{,1..3} (4 alike) : Mux  Inputs=2
  Only pos : Saturate  UpperLimit=inf  LowerLimit=0.1
  Pnt_egyDeltaChem Bat [kWh] : Display
      settings: Format=bank
  Pnt_egyElecBat2Hvl [kWh] : Display
      settings: Format=bank
  Pnt_egyElecHvl2Aux [kWh] : Display
      settings: Format=bank
  Pnt_egyElecHvl2Bat [kWh] : Display
      settings: Format=bank
  Product : Product
  "Scope (DeltaAltitude) " : Scope
  "Scope (mFuelCorr) " : Scope
  Scope of System : Scope  NumInputPorts=5
  Sum : Sum  Inputs=+-|
  Sum1 : Sum  Inputs=+-|
  Sum2 : Sum  Inputs=|++
  Sum3 : Sum  Inputs=|+-
  Sum4 : Sum  Inputs=|++
  convert : Gain  Gain=3600*1000000
  egyAccel [kWh] : Display
      settings: Format=bank
  egyBdy2GbxFr [kWh] : Display
      settings: Format=bank
  "egyBdy2GbxFr [kWh] " : Display
      settings: Format=bank
  egyBdy2GbxRe [kWh] : Display
      settings: Format=bank
  egyBdyBalance : Display
  egyDecel [kWh] : Display
      settings: Format=bank
  egyDownhill [kWh] : Display
      settings: Format=bank
  egyEdr2Gbx [kWh] : Display
      settings: Format=bank
  egyEdrBalance = 0 !!! : Display
  egyElecEdr2Hvl [kWh] : Display
      settings: Format=bank
  egyElecHvl2Edr [kWh] : Display
      settings: Format=bank
  egyGbx2Edr [kWh] : Display
      settings: Format=bank
  egyGbxFr2Bdy [kWh] : Display
      settings: Format=bank
  "egyGbxFr2Bdy [kWh] " : Display
      settings: Format=bank
  egyGbxFr2Ice[kWh] : Display
      settings: Format=bank
  egyGbxFrBalance = 0 !!! : Display
  egyGbxRe2Bdy [kWh] : Display
      settings: Format=bank
  egyGbxReBalance = 0 !!!1 : Display
  egyIce2GbxFr [kWh] : Display
      settings: Format=bank
  egyKin [kWh] : Display
      settings: Format=bank
  egyMechBdy2GbxRe [kWh] : Display
      settings: Format=bank
  egyMechEdr2Gbx [kWh] : Display
      settings: Format=bank
  egyMechEffGbx2Ice [kWh] : Display
      settings: Format=bank
  egyMechEffIce2Gbx [kWh] : Display
      settings: Format=bank
  egyMechGbx2Edr [kWh] : Display
      settings: Format=bank
  egyMechGbxRe2Bdy [kWh] : Display
      settings: Format=bank
  egyUphill [kWh] : Display
      settings: Format=bank
  egydeltaChemBat : Display
  egydeltaChemBat2 : Display
  heating value/3.6E6 : Gain  Gain=41E6/3.6E6
  "mFuel [kg] " : Display
  mFuelBal [kg] : Display
  tag scope: Bdy_egykWhAccelVeh=global, Bdy_egykWhDecelVeh=global, Bdy_egykWhDownhill=global, Bdy_egykWhDrvRes=global, Bdy_egykWhFricBrkFr=global, Bdy_egykWhFricBrkRe=global, Bdy_egykWhKin=global, Bdy_egykWhMechSlope=global, Bdy_egykWhUphill=global, Edr_egykWhEdrLosses=global, Edr_egykWhElecEdr2Hvl=global, Edr_egykWhElecHvl2Edr=global, Edr_egykWhMechEdr2Gbx=global, Edr_egykWhMechGbx2Edr=global, Gbx_egykWhBdy2GbxFr=global, Gbx_egykWhBdy2GbxRe=global, Gbx_egykWhGbx2BdyFr=global, Gbx_egykWhGbx2BdyRe=global, Gbx_egykWhGbxLossesFr=global, Gbx_egykWhGbxLossesRe=global, Ice_beIceMean=global, Ice_kWhChemFuel=global, Ice_kWhIceLosses=global, Ice_kWhMechEffGbx2Ice=global, Ice_kWhMechEffIce2Gbx=global, Ice_mFuelBalanceIce=global, Pnt_egykWhBatLosses=global, Pnt_egykWhDeltaChemBat=global, Pnt_egykWhElecBat2Hvl=global, Pnt_egykWhElecHvl2Aux=global, Pnt_egykWhElecHvl2Bat=global
  wires:
  [Bdy_egySlope] -> Monitor egySlope [J]/1
  [Gbx_egyGbx2BdyRe] -> Monitor egyPtrPropRe [J]/1
  [Bdy_egyKinVeh] -> Monitor egyKinVeh [J]/1
  [Bdy_egyDrvRes] -> Monitor egyDrvRes [J]/1
  [Gbx_egyBdy2GbxRe] -> Monitor egyPtrRecuRe [J]/1
  [Brk_egyBrkLossesRe] -> Monitor egyFricBrkRe [J]/1
  [Bdy_lenDeltaAlt] -> "Scope (DeltaAltitude) "/1, Monitor lenDeltaAlt [m]/1
  [Bdy_lenDrivenVeh] -> Monitor lenDrivenVeh [m]/1
  [Gbx_egyGbx2BdyRe] -> Gain/1
  Gain/1 -> Add5/1, Monitor egyPtrPropRe [kWh]/1
  Gain1/1 -> Add5/3, Monitor egyPtrRecuRe [kWh]/1
  [Gbx_egyBdy2GbxRe] -> Gain1/1
  Gain3/1 -> [Bdy_egykWhFricBrkRe], Add5/5, Monitor egyFricBrkRe [kWh]/1
  [Brk_egyBrkLossesRe] -> Gain3/1
  [Bdy_egyDrvRes] -> Gain4/1
  Gain4/1 -> [Bdy_egykWhDrvRes], Add5/7, Monitor egyDrvRes [kWh]/1
  [Bdy_egySlope] -> Gain5/1
  Gain5/1 -> [Bdy_egykWhMechSlope], Add5/8, Monitor egySlope [kWh]/1
  [Bdy_egyKinVeh] -> Gain6/1
  Gain6/1 -> [Bdy_egykWhKin], Add5/9, Monitor egyKinVeh [kWh]/1
  [Bdy_egySlope] -> Gain11/1
  [Brk_egyBrkLossesRe] -> Gain9/1
  [Gbx_egyGbx2BdyFr] -> Gain7/1
  [Bdy_egyKinVeh] -> Gain12/1
  [Gbx_egyBdy2GbxFr] -> Gain8/1
  [Bdy_egyDrvRes] -> Gain10/1
  Gain7/1 -> Divide1/1
  [Bdy_lenDrivenVeh] -> Gain13/1
  Divide1/1 -> Monitor egyconPtrPropFr [kWh/100km]/1, Sum/1
  Divide2/1 -> Monitor egyconPtrRecuFr [kWh/100km]/1, Sum/2
  Gain8/1 -> Divide2/1
  Gain9/1 -> Divide3/1
  Divide3/1 -> Monitor egyconFricBrkRe [kWh/100km]/1
  Gain10/1 -> Divide5/1
  Gain11/1 -> Divide6/1
  Divide5/1 -> Monitor egyconDrvRes [kWh/100km]/1
  Divide6/1 -> Monitor egyconSlope [kWh/100km]/1
  Divide7/1 -> Monitor egyconKinVeh [kWh/100km]/1
  Gain12/1 -> Divide7/1
  [Bdy_lenDrivenVeh] -> Gain14/1
  Gain14/1 -> Divide14/2, Divide11/2, Divide10/2, Divide13/2, Divide12/2, Divide5/2, Divide6/2, Divide7/2
  Sum/1 -> Monitor egyconPtrBalanceFr [kWh/100km]/1
  Gain15/1 -> Divide8/1
  Gain13/1 -> Divide3/2, Divide2/2, Divide4/2, Divide8/2, Divide1/2, Divide9/2
  Divide8/1 -> Sum1/2, Monitor egyconPtrRecuRe [kWh/100km]/1
  [Gbx_egyBdy2GbxRe] -> Gain15/1
  Gain2/1 -> Divide4/1
  [Gbx_egyGbx2BdyRe] -> Gain2/1
  Divide4/1 -> Sum1/1, Monitor egyconPtrPropRe [kWh/100km]/1
  Sum1/1 -> Monitor egyconPtrBalanceRe [kWh/100km]/1
  Gain16/1 -> Divide9/1
  [Brk_egyBrkLossesFr] -> Gain16/1
  Divide9/1 -> Monitor egyconFricBrkFr [kWh/100km]/1
  [Gbx_egyBdy2GbxFr] -> Gain18/1
  Gain17/1 -> Add5/2, Monitor egyPtrPropFr [kWh]/1
  [Gbx_egyGbx2BdyFr] -> Gain17/1
  Gain18/1 -> Add5/4, Monitor egyPtrRecuFr [kWh]/1
  [Gbx_egyGbx2BdyFr] -> Monitor egyPtrPropFr [J]/1
  [Gbx_egyBdy2GbxFr] -> Monitor egyPtrRecuFr [J]/1
  [Brk_egyBrkLossesFr] -> Monitor egyFricBrkFr [J]/1
  [Brk_egyBrkLossesFr] -> Gain19/1
  Gain19/1 -> [Bdy_egykWhFricBrkFr], Add5/6, Monitor egyFricBrkFr [kWh]/1
  Gain20/1 -> [Bdy_egykWhDecelVeh], Monitor egyDecelVeh [kWh]/1
  [Bdy_egyDecelVeh] -> Monitor egyDecelVeh [J]/1
  [Bdy_egyDecelVeh] -> Gain20/1
  [Bdy_egyAccelVeh] -> Monitor egyAccelVeh [J]/1
  [Bdy_egyAccelVeh] -> Gain21/1
  Gain21/1 -> [Bdy_egykWhAccelVeh], Monitor egyAccelVeh [kWh]/1
  Gain23/1 -> [Bdy_egykWhUphill], Monitor egyBdyUphill [kWh]/1
  [Bdy_egyBdyDownhill] -> Monitor egyBdyDownhill [J]/1
  [Bdy_egyBdyUphill] -> Monitor egyBdyUphill [J]/1
  Gain22/1 -> [Bdy_egykWhDownhill], Monitor egyBdyDownhill [kWh]/1
  [Bdy_egyBdyDownhill] -> Gain22/1
  [Bdy_egyBdyUphill] -> Gain23/1
  Divide10/1 -> Monitor egyconAccelVeh [kWh/100km]/1
  [Bdy_egyAccelVeh] -> Gain24/1
  Gain24/1 -> Divide10/1
  Divide11/1 -> Monitor egyconDecelVeh [kWh/100km]/1
  Gain25/1 -> Divide11/1
  [Bdy_egyDecelVeh] -> Gain25/1
  [Bdy_egyBdyUphill] -> Gain27/1
  [Bdy_egyBdyDownhill] -> Gain26/1
  Gain27/1 -> Divide12/1
  Gain26/1 -> Divide13/1
  Divide12/1 -> Monitor egyconBdyUphill [kWh/100km]/1
  Divide13/1 -> Monitor egyconBdyDownhill [kWh/100km]/1
  [Edr_egyElecHvl2Edr] -> Gain30/1
  [Edr_egyElecEdr2Hvl] -> Monitor egyElecEdr2Hvl [J]/1
  [Edr_egyElecHvl2Edr] -> Monitor egyElecHvl2Edr [J]/1
  Gain30/1 -> Add2/2, [Edr_egykWhElecHvl2Edr], Add1/2, Monitor egyElecHvl2Edr [kWh]/1
  Gain32/1 -> Monitor egyBatLosses [kWh]/1, [Pnt_egykWhBatLosses], Add/3, Add1/4
  [Pnt_egyBatLosses] -> Monitor egyBatLosses [J]/1
  [Pnt_egyBatLosses] -> Gain32/1
  [Pnt_egyElecHvl2Aux] -> Gain33/1
  Gain33/1 -> Add1/3, [Pnt_egykWhElecHvl2Aux], Monitor egyElecHvl2Aux [kWh]/1
  [Edr_egyMechGbx2Edr] -> Gain29/1
  Gain28/1 -> [Edr_egykWhMechEdr2Gbx], Add4/4, Add2/3, Monitor egyMechEdrProp [kWh]/1
  [Edr_egyElecEdr2Hvl] -> Gain31/1
  [Edr_egyMechEdr2Gbx] -> Gain28/1
  [Edr_egyMechEdr2Gbx] -> Monitor egyMechEdrProp [J]/1
  [Edr_egyMechGbx2Edr] -> Monitor egyMechEdrRecu [J]/1
  [Pnt_egyElecHvl2Aux] -> Monitor egyElecHvl2Aux [J]/1
  [Pnt_egyElecHvl2Bat] -> Gain34/1
  [Pnt_egyElecHvl2Bat] -> Monitor egyElecHvl2Bat [J]/1
  [Pnt_egyElecBat2Hvl] -> Gain35/1
  Gain34/1 -> Monitor egyElecHvl2Bat [kWh]/1, [Pnt_egykWhElecHvl2Bat], Add/1
  Gain35/1 -> Monitor egyElecBat2Hvl [kWh]/1, [Pnt_egykWhElecBat2Hvl], Add/2
  [Pnt_egyElecBat2Hvl] -> Monitor egyElecBat2Hvl [J]/1
  Add/1 -> [Pnt_egykWhDeltaChemBat], egydeltaChemBat/1
  Add1/1 -> egydeltaChemBat2/1
  [Edr_egyEdrLosses] -> Gain36/1
  [Edr_egyEdrLosses] -> Monitor egyEdrLosses [J]/1
  Gain36/1 -> [Edr_egykWhEdrLosses], Add2/5, Monitor egyEdrLosses [kWh]/1
  Gain29/1 -> [Edr_egykWhMechGbx2Edr], Add4/5, Add2/1, Monitor egyMechEdrRecu [kWh]/1
  Gain31/1 -> Add2/4, Monitor egyElecEdr2Hvl [kWh]/1, [Edr_egykWhElecEdr2Hvl], Add1/1
  Add2/1 -> egyEdrBalance = 0 !!!/1
  [Gbx_egyGbx2BdyRe] -> Monitor egyGbx2BdyRe [J]/1
  [Gbx_egyGbx2BdyRe] -> Gain37/1
  Gain37/1 -> [Gbx_egykWhGbx2BdyRe], Add4/1, Monitor egyGbx2BdyRe [kWh]/1
  [Gbx_egyGbx2BdyFr] -> Gain41/1
  [Gbx_egyBdy2GbxRe] -> Gain40/1
  [Gbx_egyBdy2GbxFr] -> Gain42/1
  [Gbx_egyBdy2GbxFr] -> Monitor egyBdy2GbxFr [J]/1
  Gain41/1 -> Add3/1, [Gbx_egykWhGbx2BdyFr], Monitor egyGbx2BdyFr [kWh]/1
  [Gbx_egyGbx2BdyFr] -> Monitor egyGbx2BdyFr [J]/1
  Gain40/1 -> [Gbx_egykWhBdy2GbxRe], Add4/2, Monitor egyBdy2GbxRe [kWh]/1
  [Gbx_egyBdy2GbxRe] -> Monitor egyBdy2GbxRe [J]/1
  Gain42/1 -> Add3/2, [Gbx_egykWhBdy2GbxFr], Monitor egyBdy2GbxFr [kWh]/1
  [Gbx_egyGbxLossesRe] -> Monitor egyGbxLossesRe [J]/1
  Gain43/1 -> [Gbx_egykWhGbxLossesRe], Add4/3, Monitor egyGbxLossesRe [kWh]/1
  [Gbx_egyGbxLossesRe] -> Gain43/1
  Gain44/1 -> Add3/3, [Gbx_egykWhGbxLossesFr], Monitor egyGbxLossesFr [kWh]/1
  [Gbx_egyGbxLossesFr] -> Gain44/1
  [Gbx_egyGbxLossesFr] -> Monitor egyGbxLossesFr [J]/1
  Add3/1 -> egyGbxFrBalance = 0 !!!/1
  Add4/1 -> egyGbxReBalance = 0 !!!1/1
  Ground/1 -> Add3/5, Add3/4
  Add5/1 -> egyBdyBalance/1
  [Bdy_kmhVeh] -> Mux/2
  [Pnt_facSocBat] -> Scope of System/4  "Pnt_facSocBat"
  Mux/1 -> Scope of System/1
  [Env_kmhVehDes] -> Mux/1
  [Bdy_tqBrkAxRe] -> Mux1/1
  [Edr_nEdr] -> Mux3/1  "Edr_nEdr"
  Mux1/1 -> Scope of System/2
  [Bdy_tqBrkAxFr] -> Mux1/2
  [Pnt_egykWhElecHvl2Aux] -> Pnt_egyElecHvl2Aux [kWh]/1
  [Bdy_egykWhKin] -> egyKin [kWh]/1
  [Edr_egykWhEdrLosses] -> Edr_egyEdrLosses [kWh]/1
  [Edr_egykWhMechEdr2Gbx] -> egyMechEdr2Gbx [kWh]/1
  [Pnt_egykWhElecHvl2Bat] -> Pnt_egyElecHvl2Bat [kWh]/1
  [Bdy_egykWhDrvRes] -> Bdy_egyDrvRes [kWh]/1
  [Edr_egykWhMechGbx2Edr] -> egyGbx2Edr [kWh]/1
  [Pnt_egykWhElecBat2Hvl] -> Pnt_egyElecBat2Hvl [kWh]/1
  [Pnt_egykWhBatLosses] -> Edr_egykWhBatLosses [kWh]/1
  [Gbx_egykWhGbxLossesRe] -> Gbx_egyGbxLossesRe [kWh]/1
  [Bdy_egykWhFricBrkFr] -> Bdy_egyFricBrkFr [kWh]/1
  [Gbx_egykWhBdy2GbxRe] -> egyMechBdy2GbxRe [kWh]/1
  [Edr_egykWhElecEdr2Hvl] -> egyElecEdr2Hvl [kWh]/1
  [Gbx_egykWhBdy2GbxRe] -> egyBdy2GbxRe [kWh]/1
  [Edr_egykWhMechGbx2Edr] -> egyMechGbx2Edr [kWh]/1
  [Edr_egykWhMechEdr2Gbx] -> egyEdr2Gbx [kWh]/1
  [Gbx_egykWhGbx2BdyRe] -> egyMechGbxRe2Bdy [kWh]/1
  [Edr_egykWhElecHvl2Edr] -> egyElecHvl2Edr [kWh]/1
  [Bdy_egykWhUphill] -> egyUphill [kWh]/1
  [Pnt_egykWhDeltaChemBat] -> Pnt_egyDeltaChem Bat [kWh]/1
  [Gbx_egykWhGbx2BdyRe] -> egyGbxRe2Bdy [kWh]/1
  [Bdy_egykWhFricBrkRe] -> Bdy_egyFricBrkRe [kWh]/1
  [Pnt_egykWhDeltaChemBat] -> Product/2, Divide14/1
  Divide14/1 -> Monitor egyconDeltaChemBat [kWh/100km]/1
  [Bdy_egykWhAccelVeh] -> egyAccel [kWh]/1
  [Bdy_egykWhDownhill] -> egyDownhill [kWh]/1
  [Ice_egyMechIce2Gbx] -> Gain38/1
  Gain38/1 -> [Ice_kWhMechEffIce2Gbx], Monitor egyMechIce2Gbx [kWh]/1
  [Ice_egyMechGbx2Ice] -> Gain39/1
  Gain39/1 -> Monitor egyMechGbx2Ice [kWh]/1, [Ice_kWhMechEffGbx2Ice]
  [Ice_mFuelIce] -> Ice_mFuelIce[kg]/1, convert/1, heating value/3.6E6/1
  Divide15/1 -> [Ice_beIceMean], Ice_beAverage[g/kWh]/1
  convert/1 -> Divide15/1
  Only pos/1 -> Divide15/2
  [Ice_egyMechEffIce] -> Only pos/1, Gain45/1, Ice_egyMechEffIce[J]/1
  0.25 kg/kWh/1 -> Product/1
  Product/1 -> Monitor mDeltaFuelChemBat [kg]/1, Sum2/2
  Gain45/1 -> Ice_egyMechEffIce[kWh]/1
  [Ice_mFuelIce] -> Sum2/1
  Sum2/1 -> "Scope (mFuelCorr) "/1, [Ice_mFuelBalanceIce], Monitor mFuelBalance [kg]/1
  [Ice_kWhMechEffIce2Gbx] -> egyMechEffIce2Gbx [kWh]/1
  [Ice_kWhMechEffGbx2Ice] -> egyMechEffGbx2Ice [kWh]/1
  [Ice_kWhMechEffIce2Gbx] -> egyIce2GbxFr [kWh]/1
  [Ice_kWhMechEffGbx2Ice] -> egyGbxFr2Ice[kWh]/1
  [Ice_mFuelIce] -> "mFuel [kg] "/1
  [Ice_mFuelBalanceIce] -> mFuelBal [kg]/1
  heating value/3.6E6/1 -> [Ice_kWhChemFuel], Monitor egyFuel[kWh]/1
  Mux2/1 -> Scope of System/3
  [Bdy_tqGbxAxRe] -> Mux2/1  "Bdy_tqGbxAxRe"
  [Bdy_tqGbxAxFr] -> Mux2/2  "Bdy_tqGbxAxFr"
  [Bdy_egykWhDecelVeh] -> egyDecel [kWh]/1
  [Ice_kWhIceLosses] -> Ice_egykWhIceLosses [kWh]/1
  [Gbx_egykWhGbxLossesFr] -> Gbx_egyGbxLossesFr [kWh]/1
  [Ice_kWhChemFuel] -> Ice_kWhChemFuel[kWh]/1
  [Ice_kWhChemFuel] -> Sum3/1
  [Ice_kWhMechEffIce2Gbx] -> Sum3/2
  Sum3/1 -> Sum4/1
  Sum4/1 -> [Ice_kWhIceLosses]
  [Ice_kWhMechEffGbx2Ice] -> Sum4/2
  [Gbx_egykWhBdy2GbxFr] -> egyBdy2GbxFr [kWh]/1
  [Gbx_egykWhGbx2BdyFr] -> egyGbxFr2Bdy [kWh]/1
  [Gbx_egykWhBdy2GbxFr] -> "egyBdy2GbxFr [kWh] "/1
  [Gbx_egykWhGbx2BdyFr] -> "egyGbxFr2Bdy [kWh] "/1
  [Ice_beIceMean] -> Ice_beMean[g/kWh]/1
  Mux3/1 -> Scope of System/5
  [Ice_nIce] -> Mux3/2  "Ice_nIce"

== system Model_GBXCluctchOpt_V5/Env (Environment) ==
  note: Environment Model (Env_02)
  Bdy_Bus : Inport
  "  facSlope(len) WLTC " : Lookup_n-D  NumberOfTableDimensions=1  BreakpointsForDimension1=Env_facSlope_WLTC_CUR(:,1)  Table=Env_facSlope_WLTC_CUR(:,2)  InterpMethod=Linear Lagrange  ExtrapMethod=Clip  InternalRulePriority=Speed  RndMeth=Simplest
  %2fac : Gain  Gain=0.01
  "%2fac " : Gain  Gain=0.01
  Bus Creator : BusCreator  Inputs=2
  Bus Selector1 : BusSelector  OutputSignals=Bdy_lenDrivenVeh
  "Clock " : Clock
  Constant : Constant  Value=0
  "DesiredVelocity(t) WLTC 1800 sec " : Lookup_n-D  NumberOfTableDimensions=1  BreakpointsForDimension1=Env_vVehTime_WLTC_s  Table=Env_vVehDes_WLTC_kmh  InterpMethod=Cubic spline  ExtrapMethod=Clip  InternalRulePriority=Speed  RndMeth=Simplest
  DesiredVelocity(t) NEDC 1200 sec : Lookup_n-D  NumberOfTableDimensions=1  BreakpointsForDimension1=Env_vVehTime_NEDC_s  Table=Env_vVehDes_NEDC_kmh  InterpMethod=Cubic spline  ExtrapMethod=Clip  InternalRulePriority=Speed  RndMeth=Simplest
  Env_facSlopeBAB185_CUR = f(SimTime) : Lookup  InputValues=Env_facSlopeBAB185_CUR(:,1)  Table=Env_facSlopeBAB185_CUR(:,2)  LookUpMeth=Interpolation-Use End Values  SaturateOnIntegerOverflow=off
  Env_facSlopeCrossCountry_CUR = f(SimTime) : Lookup  InputValues=Env_facSlopeCrossCountry_CUR(:,1)  Table=Env_facSlopeCrossCountry_CUR(:,2)  LookUpMeth=Interpolation-Use End Values  SaturateOnIntegerOverflow=off
  "Env_kmhDesBAB185_CUR_552s " : Lookup_n-D  NumberOfTableDimensions=1  BreakpointsForDimension1=Env_kmhDesBAB185_CUR(:,1)  Table=Env_kmhDesBAB185_CUR(:,2)  InterpMethod=Cubic spline  ExtrapMethod=Clip  InternalRulePriority=Speed  RndMeth=Simplest
  "Env_kmhDesCrossCountry_CUR_1200s " : Lookup_n-D  NumberOfTableDimensions=1  BreakpointsForDimension1=Env_kmhDesCrossCountry_CUR(:,1)  Table=Env_kmhDesCrossCountry_CUR(:,2)  InterpMethod=Cubic spline  ExtrapMethod=Clip  InternalRulePriority=Speed  RndMeth=Simplest
  Filter : Subsystem
  Goto : Goto  TagVisibility=global
  StepSpeed Down : Step  Time=150  After=-260  SampleTime=0
  StepSpeed Up : Step  Time=0  After=260  SampleTime=0
  Sum4 : Sum  Inputs=++|
  Terminator1 : Terminator
  Terminator2 : Terminator
  Terminator3 : Terminator
  facActivateSlope : Gain  Gain=-1
  Env_Bus : Outport  VectorParamsAs1DForOutWhenUnconnected=off
  tag scope: Env_kmhVehDes=global
  wires:
  Bus Creator/1 -> Env_Bus/1
  Bdy_Bus/1 -> Bus Selector1/1
  Filter/1(out) -> [Env_kmhVehDes], Bus Creator/1  "Env_kmhVehDes"
  Bus Selector1/1 -> "  facSlope(len) WLTC "/1  "<Bdy_lenDrivenVeh>"
  "Clock "/1 -> Env_facSlopeCrossCountry_CUR = f(SimTime)/1, Env_facSlopeBAB185_CUR = f(SimTime)/1, "Env_kmhDesCrossCountry_CUR_1200s "/1, "Env_kmhDesBAB185_CUR_552s "/1, DesiredVelocity(t) NEDC 1200 sec/1, "DesiredVelocity(t) WLTC 1800 sec "/1
  "Env_kmhDesBAB185_CUR_552s "/1 -> Terminator1/1, Filter/1(in)  "Env_kmhVehDes [km/h]"
  facActivateSlope/1 -> Goto/1, Bus Creator/2  "Env_facSlope"
  StepSpeed Up/1 -> Sum4/2
  StepSpeed Down/1 -> Sum4/1
  Sum4/1 -> Terminator2/1
  Constant/1 -> Terminator3/1  "Env_facSlope"
  Env_facSlopeBAB185_CUR = f(SimTime)/1 -> %2fac/1
  Env_facSlopeCrossCountry_CUR = f(SimTime)/1 -> "%2fac "/1
  %2fac/1 -> facActivateSlope/1

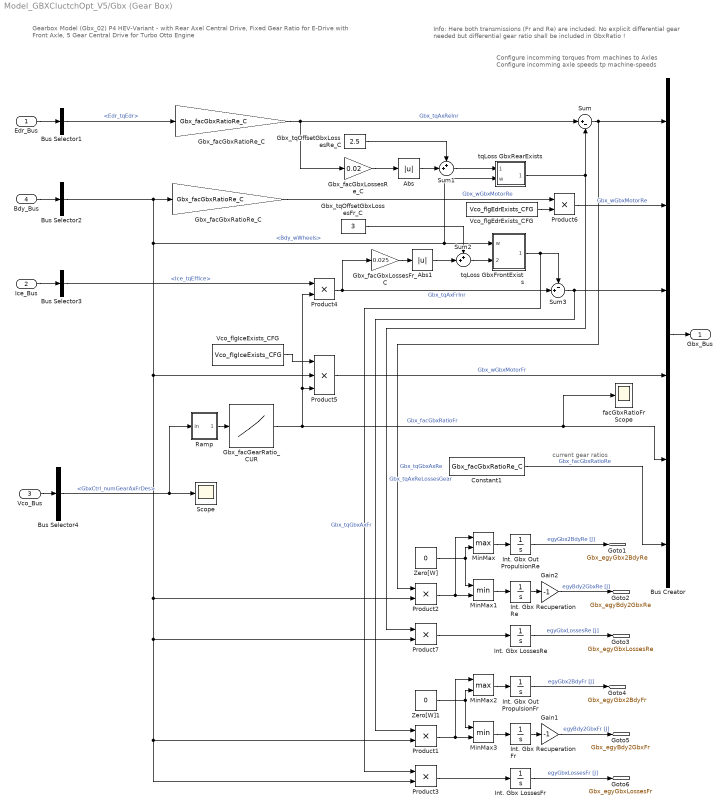
== system Model_GBXCluctchOpt_V5/Gbx (Gear Box) ==
  note: Info:
      | Here both transmissions (Fr and Re) are included. No explicit differential gear needed but differential gear ratio shall be included in GbxRatio !
  note: current gear ratios
  note: Configure incomming torques from machines to Axles
      | Configure incomming axle speeds tp machine-speeds
  note: Gearbox Model (Gbx_02)
      | P4 HEV-Variant - with Rear Axel Central Drive, Fixed Gear Ratio for E-Drive
      | with Front Axle, 5 Gear Central Drive for Turbo Otto Engine
  Edr_Bus : Inport
  Ice_Bus : Inport  Port=2
  Vco_Bus : Inport  Port=3
  Bdy_Bus : Inport  Port=4
  Abs : Abs  SaturateOnIntegerOverflow=off
  Abs1 : Abs  SaturateOnIntegerOverflow=off
  Bus Creator : BusCreator  Inputs=6
  Bus Selector1 : BusSelector  OutputSignals=Edr_tqEdr
  Bus Selector2 : BusSelector  OutputSignals=Bdy_wWheels
  Bus Selector3 : BusSelector  OutputSignals=Ice_tqEffIce
  Bus Selector4 : BusSelector  OutputSignals=GbxCtrl_numGearAxFrDes
  Constant1 : Constant  Value=Gbx_facGbxRatioRe_C
  Gain1 : Gain  Gain=-1
  Gain2 : Gain  Gain=-1
  Gbx_facGbxLossesFr_C : Gain  Gain=0.025
  Gbx_facGbxLossesRe_C : Gain  Gain=0.02
  Gbx_facGbxRatioRe_C : Gain  Gain=Gbx_facGbxRatioRe_C
  "Gbx_facGbxRatioRe_C " : Gain  Gain=Gbx_facGbxRatioRe_C
  "Gbx_facGearRatio_CUR " : Lookup_n-D  NumberOfTableDimensions=1  BreakpointsForDimension1="[1 2  3  4   5]"  Table="[10 7.1 5  3.6  2.6 ]"  ExtrapMethod=Clip  InternalRulePriority=Speed  RndMeth=Simplest
  Gbx_tqOffsetGbxLossesFr_C : Constant  Value=3
  Gbx_tqOffsetGbxLossesRe_C : Constant  Value=2.5
  Int. Gbx LossesFr : Integrator
  Int. Gbx LossesRe : Integrator
  Int. Gbx Out PropulsionFr : Integrator
  Int. Gbx Out PropulsionRe : Integrator
  Int. Gbx RecuperationFr : Integrator
  Int. Gbx RecuperationRe : Integrator
  MinMax : MinMax  Function=max  Inputs=2  ZeroCross=off
  MinMax1 : MinMax  Inputs=2  ZeroCross=off
  MinMax2 : MinMax  Function=max  Inputs=2  ZeroCross=off
  MinMax3 : MinMax  Inputs=2  ZeroCross=off
  Product{1..4,6..7} (6 alike) : Product
  Product5 : Product  Inputs=3
  Ramp : Subsystem
  Scope : Scope
  Sum : Sum  Inputs=|+-
  Sum1 : Sum  Inputs=++|
  Sum2 : Sum  Inputs=++|
  Sum3 : Sum  Inputs=-+|
  Vco_flgEdrExists_CFG : Constant  Value=Vco_flgEdrExists_CFG
  Vco_flgIceExists_CFG : Constant  Value=Vco_flgIceExists_CFG
  Zero[W] : Constant  Value=0
  Zero[W]1 : Constant  Value=0
  facGbxRatioFr Scope : Scope
  tqLoss GbxFrontExists : Subsystem
  tqLoss GbxRearExists : Subsystem
  Gbx_Bus : Outport  VectorParamsAs1DForOutWhenUnconnected=off
  tag scope: Gbx_egyBdy2GbxFr=global, Gbx_egyBdy2GbxRe=global, Gbx_egyGbx2BdyFr=global, Gbx_egyGbx2BdyRe=global, Gbx_egyGbxLossesFr=global, Gbx_egyGbxLossesRe=global
  wires:
  Bus Creator/1 -> Gbx_Bus/1
  Sum/1 -> Bus Creator/1, Product2/1  "Gbx_tqGbxAxRe"
  Product4/1 -> Gbx_facGbxLossesFr_C/1, Sum3/2  "Gbx_tqAxFrInr"
  Edr_Bus/1 -> Bus Selector1/1
  Bus Selector1/1 -> Gbx_facGbxRatioRe_C/1  "<Edr_tqEdr>"
  "Gbx_facGbxRatioRe_C "/1 -> Product6/1  "Gbx_wGbxMotorRe"
  Product5/1 -> Bus Creator/4  "Gbx_wGbxMotorFr"
  Bdy_Bus/1 -> Bus Selector2/1
  Bus Selector2/1 -> Product2/2, Product7/2, Product1/2, Product3/2, Product5/2, tqLoss GbxRearExists/2(w), tqLoss GbxFrontExists/1(w), "Gbx_facGbxRatioRe_C "/1  "<Bdy_wWheels>"
  Ice_Bus/1 -> Bus Selector3/1
  Bus Selector3/1 -> Product4/1  "<Ice_tqEffIce>"
  "Gbx_facGearRatio_CUR "/1 -> Product4/2, Product5/3, facGbxRatioFr Scope/1, Bus Creator/5  "Gbx_facGbxRatioFr"
  Constant1/1 -> Bus Creator/6  "Gbx_facGbxRatioRe"
  Vco_Bus/1 -> Bus Selector4/1
  Bus Selector4/1 -> Scope/1, Ramp/1(in)  "<GbxCtrl_numGearAxFrDes>"
  tqLoss GbxRearExists/1(tqOut) -> Sum/2, Product7/1  "Gbx_tqAxReLossesGear"
  Abs/1 -> Sum1/2
  Gbx_facGbxLossesRe_C/1 -> Abs/1
  Gbx_facGbxRatioRe_C/1 -> Sum/1, Gbx_facGbxLossesRe_C/1  "Gbx_tqAxReInr"
  Gbx_tqOffsetGbxLossesRe_C/1 -> Sum1/1
  MinMax/1 -> Int. Gbx Out PropulsionRe/1
  Product7/1 -> Int. Gbx LossesRe/1
  MinMax1/1 -> Int. Gbx RecuperationRe/1
  Int. Gbx Out PropulsionRe/1 -> [Gbx_egyGbx2BdyRe]  "egyGbx2BdyRe [J]"
  Int. Gbx LossesRe/1 -> [Gbx_egyGbxLossesRe]  "egyGbxLossesRe [J]"
  Zero[W]/1 -> MinMax1/1, MinMax/2
  Int. Gbx RecuperationRe/1 -> Gain2/1
  Product2/1 -> MinMax/1, MinMax1/2
  Gain2/1 -> [Gbx_egyBdy2GbxRe]  "egyBdy2GbxRe [J]"
  Sum1/1 -> tqLoss GbxRearExists/1(tqIn)
  Zero[W]1/1 -> MinMax3/1, MinMax2/2
  Int. Gbx RecuperationFr/1 -> Gain1/1
  Int. Gbx LossesFr/1 -> [Gbx_egyGbxLossesFr]  "egyGbxLossesFr [J]"
  Int. Gbx Out PropulsionFr/1 -> [Gbx_egyGbx2BdyFr]  "egyGbx2BdyFr [J]"
  MinMax3/1 -> Int. Gbx RecuperationFr/1
  Product1/1 -> MinMax2/1, MinMax3/2
  MinMax2/1 -> Int. Gbx Out PropulsionFr/1
  Product3/1 -> Int. Gbx LossesFr/1
  Gain1/1 -> [Gbx_egyBdy2GbxFr]  "egyBdy2GbxFr [J]"
  tqLoss GbxFrontExists/1(tqOut) -> Product3/1, Sum3/1
  Ramp/1(Out) -> "Gbx_facGearRatio_CUR "/1
  Sum3/1 -> Bus Creator/3, Product1/1  "Gbx_tqGbxAxFr"
  Sum2/1 -> tqLoss GbxFrontExists/2(tqIn)
  Gbx_tqOffsetGbxLossesFr_C/1 -> Sum2/1
  Gbx_facGbxLossesFr_C/1 -> Abs1/1
  Abs1/1 -> Sum2/2
  Vco_flgIceExists_CFG/1 -> Product5/1
  Product6/1 -> Bus Creator/2  "Gbx_wGbxMotorRe"
  Vco_flgEdrExists_CFG/1 -> Product6/2
